simulink library "xpcseriallib"  (Simulink 7.7)
settings: Solver=FixedStepDiscrete  StartTime=0.0  StopTime=inf  RelTol=1e-3
undefined symbols (not defined in the file or in its folder): baddr1, baddr2, mbaseserialbinmask, mbaseserialmask, mdiamondemeraldfifomask, mdiamondemeraldmask, mmodemcontrol, mqua2mask, mquafifomask, mquamask, mrs232
libraries: xpcseriallib x614, xpclib x16, simulink x12
(part 1 of 7)
settings Model: Creator=gweast  LastModifiedBy=Darryl

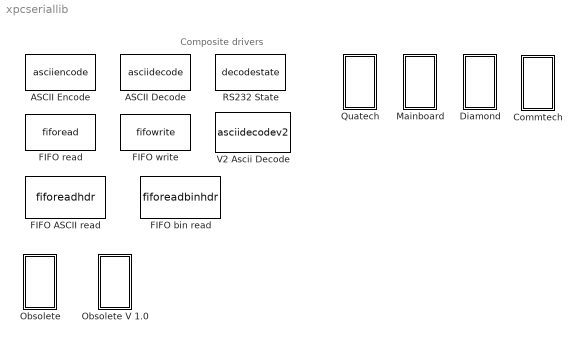
== system xpcseriallib ==
  note: Composite drivers
  "ASCII Decode " : S-Function  FunctionName=asciidecode  Parameters=format, nvars, varids  EnableBusSupport=off  mask(ASCII Decode){format=%d\\r, nvars=1, vartypes={ }}
      mask prompts: format "Format string:"; nvars "Number of variables:"; vartypes "Variable types:"
      mask help: ASCII decode -- Decode input string to output variables
      mask init:
      | [ maskdisplay, varids, format ] = masciidecode( 2, format, nvars, vartypes, 1 );
      | set_param( gcb, 'MaskDisplay', maskdisplay );
      mask Help: helpview(fullfile(docroot, 'mapfiles', 'xpc.map'), 'Quatech_ASCII_Decode')
      mask Display: disp( 'ASCII\nDecode');port_label('input',1,'D');port_label('output',1,'1');
  "ASCII Encode " : S-Function  FunctionName=asciiencode  Parameters=format, maxlength, nvars, varids  EnableBusSupport=off  mask(ASCII Encode){format=%d\\r, nvars=1, maxlength=128, vartypes={ 'double' }}
      mask prompts: format "Format string:"; nvars "Number of variables:"; maxlength "Max output string length:"; vartypes "Variable types:"
      mask help: ASCII Encode -- encode input variables as ascii for RS232.
      mask init:
      | [ maskdisplay, varids, format ] = masciidecode( 2, format, nvars, vartypes, 2 );
      | set_param( gcb, 'MaskDisplay', maskdisplay );
      mask Help: helpview(fullfile(docroot, 'mapfiles', 'xpc.map'), 'Quatech_ASCII_Encode')
      mask Display: disp( 'ASCII\nEncode');port_label('output',1,'D');port_label('input',1,'1');
  Commtech : Subsystem
      settings: OpenFcn=load_open_subsystem('xpccommtechlib',['xpccommtechlib/RS-422 &',char(10),'RS-485']);
  Diamond : Subsystem
  "FIFO ASCII read " : S-Function  FunctionName=fiforeadhdr  Parameters=maxsize, outputtype, sampletime, hdr, hlengths, nterm, hold, enable  EnableBusSupport=off  mask(Asynchronous FIFO Block: reader){header={'Header1','Header2'}, term=[13 10], hold=Zero output if no new data, enable=off, maxsize=1024, outputtype=8 bit uint null terminated, sampletime=0.01}
      mask prompts: term "Terminating string:"; hold "Output behavior:"; enable "Enable input:"; maxsize "Maximum read size:"; outputtype "Output vector type:"
      mask help: FIFO read multiple headers
      mask init:
      | [maskdisplay, hdr, hlengths, nterm] = mfiforhdr( header, term );
      | set_param( gcb, 'MaskDisplay', maskdisplay );
      mask Help: helpview(fullfile(docroot, 'mapfiles', 'xpc.map'), 'FIFO_asciiread')
      mask StyleString: edit,edit,popup(Hold last output if no new data|Zero output if no new data),checkbox,edit,popup(count+32 bit int|count+32 bit uint|count+16 bit int|count+16 bit uint|8 bit int null terminated|8 bit uint null terminated),edit
      mask Display: disp( 'FIFO\nRead HDRS');port_label('input',1,'F');port_label('output',1,'1');port_label('output',2,'2');
  "FIFO bin read " : S-Function  FunctionName=fiforeadbinhdr  Parameters=maxsize, outputtype, sampletime, hdr, hlengths, lengths, hold, enable  EnableBusSupport=off  mask(Asynchronous FIFO Block: reader){header={char([170, 1]), char([170,2])}, lengths=[3 4], hold=Zero output if no new data, enable=off, maxsize=1024, outputtype=8 bit uint null terminated, sampletime=0.01}
      mask prompts: lengths "Message Lengths:"; hold "Output behavior:"; enable "Enable input:"; maxsize "Maximum read size:"; outputtype "Output vector type:"
      mask help: FIFO read multiple binary headers
      mask init:
      | [maskdisplay, hdr, hlengths] = mfifobinhdr( header, lengths );
      | set_param( gcb, 'MaskDisplay', maskdisplay );
      mask Help: helpview(fullfile(docroot, 'mapfiles', 'xpc.map'), 'FIFO_binread')
      mask StyleString: edit,edit,popup(Hold last output if no new data|Zero output if no new data),checkbox,edit,popup(count+32 bit int|count+32 bit uint|count+16 bit int|count+16 bit uint|8 bit int null terminated|8 bit uint null terminated),edit
      mask Display: disp( 'FIFO\nRead BINARY');port_label('input',1,'F');port_label('output',1,'1');port_label('output',2,'2');
  "FIFO read " : S-Function  FunctionName=fiforead  Parameters=maxsize, minsize, usedelimiter, delimiter, outputtype, sampletime, enable, enableout  EnableBusSupport=off  mask(Asynchronous FIFO Block: reader){maxsize=1024, minsize=1, usedelimiter=on, delimiter=13, outputtype=8 bit uint null terminated, enable=off, enableout=off, sampletime=0.001}
      mask prompts: maxsize "Maximum read size:"; minsize "Minimum read size:"; usedelimiter "Read to delimiter:"; outputtype "Output vector type:"; enable "Max and Min read size ports:"; enableout "Enable passthrough:"
      mask help: FIFO read
      mask init:
      | maskdisplay = mfiforw( enable, enableout, 2 );
      | set_param( gcb, 'MaskDisplay', maskdisplay );
      mask Help: helpview(fullfile(docroot, 'mapfiles', 'xpc.map'), 'Quatech_FIFO_Read')
      mask StyleString: edit,edit,checkbox,edit,popup(count+32 bit int|count+32 bit uint|count+16 bit int|count+16 bit uint|8 bit int null terminated|8 bit uint null terminated),checkbox,checkbox,edit
      mask Display: disp( 'FIFO\nRead');port_label('output',1,'D');port_label('input',1,'F');
  "FIFO write " : S-Function  FunctionName=fifowrite  Parameters=size, inputtype, sampletime, present, id  EnableBusSupport=off  mask(Asynchronous FIFO Block: writer){size=1024, inputtype=8 bit uint null terminated, present=off, sampletime=-1, id=}
      mask prompts: inputtype "Input vector type:"; present "Data present output:"; id "ID (for overflow messages):"
      mask help: FIFO write
      mask init:
      | maskdisplay = mfiforw( present, 0, 1 );
      | set_param(gcb,'MaskDisplay',maskdisplay);
      mask Help: helpview(fullfile(docroot, 'mapfiles', 'xpc.map'), 'Quatech_FIFO_Write')
      mask StyleString: edit,popup(count+32 bit int|count+32 bit uint|count+16 bit int|count+16 bit uint|8 bit int null terminated|8 bit uint null terminated),checkbox,edit,edit
      mask Display: disp( 'FIFO\nwrite');port_label('input',1,'D');port_label('output', 1, 'F');
  Mainboard : Subsystem
  Obsolete : Subsystem
  Obsolete V 1.0 : Subsystem
  Quatech : Subsystem
  RS232 State : S-Function  FunctionName=decodestate  Parameters=overrun, parity, frame, breakint, count  EnableBusSupport=off  mask(RS232 State){overrun=on, parity=on, frame=off, breakint=off}
      mask prompts: overrun "Overrun error output:"; parity "Parity error output"; frame "Framing error output"; breakint "Break interrupt output"
      mask help: RS232 State
      mask init:
      | count = 0;
      | [maskdisplay, count] = mdecodestate( overrun, parity, frame, breakint );
      | set_param( gcb, 'MaskDisplay', maskdisplay );
      mask Help: helpview(fullfile(docroot, 'mapfiles', 'xpc.map'), 'Quatech_State')
      mask Display: disp('RS232\nState');port_label('input',1,'D');port_label('output',1,'D');port_label('output',2,'O');port_label('output',3,'P');
  "V2 Ascii Decode " : S-Function  FunctionName=asciidecodev2  Parameters=format, types  EnableBusSupport=off  mask(asciidecode2){format='%f\\n'}
      mask help: ASCII decode
      mask init:
      | [maskdisplay, types] = masciidecodev2( format );
      | set_param( gcb, 'MaskDisplay', maskdisplay );
      mask Help: helpview(fullfile(docroot, 'mapfiles', 'xpc.map'), 'ASCII_Decode2')
      mask Display: disp('Ascii Decode\nV2');port_label('output',1,'cnt');

== system xpcseriallib/Commtech ==

== system xpcseriallib/Diamond ==
  "Emerald-MM " : Subsystem
  "Emerald-MM8 " : Subsystem

== system xpcseriallib/Mainboard ==
  Baseboard Serial : Subsystem  InitFcn=mbaseserialmask(4,2);  mask(Baseboard RS232 Send Receive){group=Board Setup, port=1, irqnum=4, saddr1=0x3f8, saddr2=0x3e8, config=Com1/none, baud1=115200, parity1=None, ndata1=8, nstop1=1, fifomode1=16 deep, rlevel1=half full, automode1=off, xmtfifosize1=1024, xmtdatatype1=8 bit uint null terminated, rcvfifosize1=1024, rcvmaxread1=1024, rcvminread1=1, rcvusedelim1=on, rcvdelim1=13, rcvdatatype1=count+16 bit uint, rcvsampletime1=.01, baud2=115200, parity2=None, ndata2=8, nstop2=1, fifomode2=16 deep, rlevel2=half full, automode2=off, xmtfifosize2=1024, xmtdatatype2=8 bit uint null terminated, rcvfifosize2=1024, rcvmaxread2=1024, rcvminread2=1, rcvusedelim2=on, rcvdelim2=13, rcvdatatype2=count+16 bit uint, rcvsampletime2=.01}
      mask prompts: group "Parameter group:"; port "Port to modify:"; irqnum "IRQ number:"; saddr1 "First port address:"; saddr2 "Second port address:"; config "Configuration:"; baud1 "Baud rate:"; parity1 "Parity:"; ndata1 "Data bits:"; nstop1 "Stop bits:"; fifomode1 "Hardware FIFO size:"; rlevel1 "Receive FIFO interrupt level:"; automode1 "Auto RTS/CTS:"; xmtfifosize1 "Transmit software FIFO size:"; xmtdatatype1 "Transmit FIFO data type:"; rcvfifosize1 "Receive software FIFO size:"; rcvmaxread1 "Receive maximum read:"; rcvminread1 "Receive minimum read:"; rcvusedelim1 "Read to delimiter:"; rcvdelim1 "Delimiter:"; rcvdatatype1 "Receive data type:"; rcvsampletime1 "Receive SampleTime:"; baud2 "Baud rate:"; parity2 "Parity:"; ndata2 "Data bits:"; nstop2 "Stop bits:"; fifomode2 "Hardware FIFO size:"; rlevel2 "Receive FIFO interrupt level:"; automode2 "Auto RTS/CTS:"; xmtfifosize2 "Transmit software FIFO size:"; xmtdatatype2 "Transmit FIFO data type:"; rcvfifosize2 "Receive software fifo size:"; rcvmaxread2 "Receive maximum read:"; rcvminread2 "Receive minimum read:"; rcvusedelim2 "Read to delimiter:"; rcvdelim2 "Delimiter:"; rcvdatatype2 "Receive data type:"; rcvsampletime2 "Receive SampleTime:"
      mask help:
      | Baseboard
      | RS232 Send Receive Subsystem
      mask init:
      | [addr1, addr2, maskdisplay] = mbaseserialmask( 1, 2 );
      | baddr1 = addr1;
      | baddr2 = addr2;
      | mbaseserialmask( 3, 2 );
      | set_param( gcb, 'MaskDisplay', maskdisplay );
      mask Help: helpview(fullfile(docroot, 'mapfiles', 'xpc.map'), 'Baseboard_Serial_Subsystem')
      mask StyleString: popup(Board Setup|Basic Setup|Transmit Setup|Receive Setup),popup(1|2),edit,edit,edit,popup(Com1/none|Com2/none|Com1/Com3|Com2/Com4|none/Com3|none/Com4|Custom),popup(115200|57600|38400|19200|9600|4800|2400|1200|600|300|110),popup(None|Even|Odd|Mark|Space),popup(5|6|7|8),popup(1|2),popup(64 deep|16 deep|1 deep),popup(1|quarter full|half full|almost full),checkbox,edit,popup(count+32 bit int|count+32 bit uint|count+16 bit int|count+16 bit uint|8 bit int null terminated|8 bit uint null terminated),edit,edit,edit,checkbox,edit,popup(count+32 bit int|count+32 bit uint|count+16 bit int|count+16 bit uint|8 bit int null terminated|8 bit uint null terminated),edit,popup(115200|57600|38400|19200|9600|4800|2400|1200|600|300|110),popup(None|Even|Odd|Mark|Space),popup(5|6|7|8),popup(1|2),popup(64 deep|16 deep|1 deep),popup(1|quarter full|half full|almost full),checkbox,edit,popup(count+32 bit int|count+32 bit uint|count+16 bit int|count+16 bit uint|8 bit int null terminated|8 bit uint null terminated),edit,edit,edit,checkbox,edit,popup(count+32 bit int|count+32 bit uint|count+16 bit int|count+16 bit uint|8 bit int null terminated|8 bit uint null terminated),edit
      mask CallbackString:
      | mbaseserialmask( 2, 2 );
      | |mbaseserialmask( 2, 2 );||||mbaseserialmask( 2, 2 );
      | ||||||||||||||||||||||||||||||||
      mask Display: disp('Baseboard\nRS232\nSend Receive');port_label('input',1,'XMT1');port_label('input',2,'');port_label('output',1,'RCV1');port_label('output',2,'');
  Baseboard Serial Internal  blocks : Subsystem
  Baseboard Serial F : Subsystem  InitFcn=mbaseserialbinmask(4,2);  mask(Baseboard RS232 Send Receive){group=Board Setup, port=1, irqnum=4, saddr1=0x3f8, saddr2=0x3e8, config=Com1/none, baud1=115200, parity1=None, ndata1=8, nstop1=1, fifomode1=16 deep, rlevel1=half full, automode1=off, xmtfifosize1=1024, xmtdatatype1=8 bit uint null terminated, rcvfifosize1=1024, baud2=115200, parity2=None, ndata2=8, nstop2=1, fifomode2=16 deep, rlevel2=half full, automode2=off, xmtfifosize2=1024, xmtdatatype2=8 bit uint null terminated, rcvfifosize2=1024}
      mask prompts: group "Parameter group:"; port "Port to modify:"; irqnum "IRQ number:"; saddr1 "First port address:"; saddr2 "Second port address:"; config "Configuration:"; baud1 "Baud rate:"; parity1 "Parity:"; ndata1 "Data bits:"; nstop1 "Stop bits:"; fifomode1 "Hardware FIFO size:"; rlevel1 "Receive FIFO interrupt level:"; automode1 "Auto RTS/CTS:"; xmtfifosize1 "Transmit software FIFO size:"; xmtdatatype1 "Transmit FIFO data type:"; rcvfifosize1 "Receive software FIFO size:"; baud2 "Baud rate:"; parity2 "Parity:"; ndata2 "Data bits:"; nstop2 "Stop bits:"; fifomode2 "Hardware FIFO size:"; rlevel2 "Receive FIFO interrupt level:"; automode2 "Auto RTS/CTS:"; xmtfifosize2 "Transmit software FIFO size:"; xmtdatatype2 "Transmit FIFO data type:"; rcvfifosize2 "Receive software fifo size:"
      mask help:
      | Baseboard
      | RS232 Send Receive Subsystem
      mask init:
      | [addr1, addr2, maskdisplay] = mbaseserialbinmask( 1, 2 );
      | baddr1 = addr1;
      | baddr2 = addr2;
      | mbaseserialbinmask( 3, 2 );
      | set_param( gcb, 'MaskDisplay', maskdisplay );
      mask Help: helpview(fullfile(docroot, 'mapfiles', 'xpc.map'), 'Baseboard_Serial_Subsystem')
      mask StyleString: popup(Board Setup|Basic Setup|FIFO Setup),popup(1|2),edit,edit,edit,popup(Com1/none|Com2/none|Com1/Com3|Com2/Com4|none/Com3|none/Com4|Custom),popup(115200|57600|38400|19200|9600|4800|2400|1200|600|300|110),popup(None|Even|Odd|Mark|Space),popup(5|6|7|8),popup(1|2),popup(64 deep|16 deep|1 deep),popup(1|quarter full|half full|almost full),checkbox,edit,popup(count+32 bit int|count+32 bit uint|count+16 bit int|count+16 bit uint|8 bit int null terminated|8 bit uint null terminated),edit,popup(115200|57600|38400|19200|9600|4800|2400|1200|600|300|110),popup(None|Even|Odd|Mark|Space),popup(5|6|7|8),popup(1|2),popup(64 deep|16 deep|1 deep),popup(1|quarter full|half full|almost full),checkbox,edit,popup(count+32 bit int|count+32 bit uint|count+16 bit int|count+16 bit uint|8 bit int null terminated|8 bit uint null terminated),edit
      mask CallbackString:
      | mbaseserialbinmask( 2, 2 );
      | |mbaseserialbinmask( 2, 2 );||||mbaseserialbinmask( 2, 2 );
      | ||||||||||||||||||||
      mask Display: disp('Baseboard\nRS232\nSend Receive\nFIFO OUT');port_label('input',1,'XMT1');port_label('input',2,'');port_label('output',1,'FIFO1');port_label('output',2,'');
  Modem Control : S-Function  InitFcn=mmodemcontrol(4)  FunctionName=modemcontrolbase  Parameters=addr, boardtype, rts, dtr, count  EnableBusSupport=off  mask(Baseboard Modem Control){rts=on, dtr=on, config=Com1, addr=0x3f8}
      mask prompts: config "Configuration:"; addr "Base address:"
      mask help:
      | Baseboard
      | Modem Control
      mask init:
      | count = 0;
      | boardtype = 4;
      | [maskdisplay, count, addr] = mmodemcontrol( 2, rts, dtr, boardtype, config, addr );
      | addr = hex2dec( addr(3:end) );
      | set_param( gcb, 'MaskDisplay', maskdisplay );
      mask Help: helpview(fullfile(docroot, 'mapfiles', 'xpc.map'), 'Baseboard_MODEM_Control')
      mask StyleString: checkbox,checkbox,popup(Com1|Com2|Com3|Com4|Custom),edit
      mask CallbackString:
      | ||mmodemcontrol( 1 );
      | |
      mask Display: disp('Baseboard\nModem Control');port_label('input',1,'RTS');port_label('input',2,'DTR');
  Modem Status : S-Function  FunctionName=modemstatusbase  Parameters=addr, boardtype, cts, dsr, ring, dcd, count, sampletime  EnableBusSupport=off  mask(Modem Status){cts=on, dsr=on, ring=on, dcd=on, sampletime=-1, config=Com1, addr=0x3f8}
      mask prompts: ring "RI:"; config "Configuration:"; addr "Base address:"
      mask help:
      | Baseboard
      | Modem Status
      mask init:
      | count = 0;
      | boardtype = 4;
      | [maskdisplay, count, addr] = mmodemstatus( 2, cts, dsr, ring, dcd, boardtype, config, addr );
      | addr = hex2dec( addr(3:end) );
      | set_param( gcb, 'MaskDisplay', maskdisplay );
      mask Help: helpview(fullfile(docroot, 'mapfiles', 'xpc.map'), 'Baseboard_MODEM_Status')
      mask StyleString: checkbox,checkbox,checkbox,checkbox,edit,popup(Com1|Com2|Com3|Com4|Custom),edit
      mask CallbackString:
      | |||||mmodemstatus( 1 );
      | |
      mask Display: disp('Baseboard\nModem Status');port_label('output',1,'CTS');port_label('output',2,'DSR');port_label('output',3,'RI');port_label('output',4,'DCD');

== system xpcseriallib/Obsolete ==
  Asynchronous Mode : Subsystem
  Binary Mode : Subsystem
  "RS232 Setup " : S-Function  InitFcn=mrs232(0);  FunctionName=rs232setup  Parameters=port, baud, dbits, sbits, parity, prot, sbuf, rbuf, 0, istr, iack, iackto, tstr, tack, tackto, initinfo, initackinfo, terminfo, termackinfo  EnableBusSupport=off  mask(rs232setup){port=COM1, baud=9600, dbits=8, sbits=1, parity=None, prot=None, sbuf=1024, rbuf=1024, initstruct=[], termstruct=[]}
      mask prompts: baud "Baud rate:"; dbits "Number of data bits:"; sbits "Number of stop bits:"; prot "Protocol:"; sbuf "Send buffer size:"; rbuf "Receive buffer size:"; initstruct "Initialization command structure:"; termstruct "Termination command structure:"
      mask help:
      | RS-232
      | Mainboard
      | Setup
      mask init:
      | dmy = '';
      | [istr,iack,dmy,maskdisplay,maskdescription,dmy,dmy,dmy,dmy,initinfo,initackinfo,iackto]=mrs232(2,initstruct,4);
      | [tstr,tack,dmy,maskdisplay,maskdescription,dmy,dmy,dmy,dmy,terminfo,termackinfo,tackto]=mrs232(1,termstruct,4);
      | set_param(gcb,'MaskDisplay',maskdisplay);
      | set_param(gcb,'MaskDescription',maskdescription);
      mask Help: helpview(fullfile(docroot, 'mapfiles', 'xpc.map'), 'RS232_RS232')
      mask StyleString: popup(COM1|COM2|COM3|COM4),popup(115200|57600|38400|19200|9600|4800|2400|1200|600|300|110),popup(8|7),popup(1|2),popup(None|Odd|Even),popup(None|XOn XOff),edit,edit,edit,edit
      mask Display: disp('RS-232\nMainboard\nSetup');
  Synchronous Mode : Subsystem

== system xpcseriallib/Obsolete V 1.0 ==
  Asynchronous Mode : Subsystem
  "Setup " : Subsystem  mask(rs232setup){port=COM2, baudrate=115200, databit=8, stopbit=1, parity=None, protocol=None, sendbuf=1024, recbuf=1024}
      mask prompts: baudrate "Baud rate:"; databit "Number of data bits:"; stopbit "Number of stop bits:"; sendbuf "Send buffer size:"; recbuf "Receive buffer size:"
      mask help:
      | RS232 Kernel resident serial driver setup (Obsolete)
      | Version 1.0 compatible for backward compatibility
      | Not for use in new models
      mask Help: helpview(fullfile(docroot,'mapfiles','xpc.map'),'RS232_Setup');
      mask StyleString: popup(COM1|COM2|COM3|COM4),popup(115200|57600|38400|19200|9600|4800|2400|1200|300|110),popup(8|7|6|5),popup(1|2),popup(None|Odd|Even),popup(None|XOnXOff|RTSCTS|DTRDSR),edit,edit
      mask Display: disp('RS232\nMainboard\nSetup');
  Synchronous Mode : Subsystem

== system xpcseriallib/Quatech ==
  DSCP-200/300 : Subsystem
  ESC-100 : Subsystem
  QSC-100 : Subsystem
  QSC-200/300 : Subsystem

== system xpcseriallib/Diamond/Emerald-MM  ==
  Diamond Emerald-MM : Subsystem
  Diamond Emerald-MM Serial : Subsystem  InitFcn=mdiamondemeraldmask(4,4);  mask(Emerald-MM RS232 Send Receive){group=Board Setup, port=1, irqnum=7, saddr1=0x240, baud1=115200  (HS 460800), parity1=None, ndata1=8, nstop1=1, fifomode1=16 deep, rlevel1=half full, automode1=on, xmtfifosize1=1024, xmtdatatype1=8 bit uint null terminated, rcvfifosize1=1024, rcvmaxread1=1024, rcvminread1=1, rcvusedelim1=on, rcvdelim1=13, rcvdatatype1=count+16 bit uint, rcvsampletime1=-1, baud2=115200  (HS 460800), parity2=None, ndata2=8, nstop2=1, fifomode2=16 deep, rlevel2=half full, automode2=on, xmtfifosize2=1024, xmtdatatype2=8 bit uint null terminated, rcvfifosize2=1024, rcvmaxread2=1024, rcvminread2=1, rcvusedelim2=on, rcvdelim2=13, rcvdatatype2=count+16 bit uint, rcvsampletime2=-1, baud3=115200  (HS 460800), parity3=None, ndata3=8, nstop3=1, fifomode3=16 deep, rlevel3=half full, automode3=on, xmtfifosize3=1024, xmtdatatype3=8 bit uint null terminated, rcvfifosize3=1024, rcvmaxread3=1024, rcvminread3=1, rcvusedelim3=on, rcvdelim3=13, rcvdatatype3=count+16 bit uint, rcvsampletime3=-1, baud4=115200  (HS 460800), parity4=None, ndata4=8, nstop4=1, fifomode4=16 deep, rlevel4=half full, automode4=on, xmtfifosize4=1024, xmtdatatype4=8 bit uint null terminated, rcvfifosize4=1024, rcvmaxread4=1024, rcvminread4=1, rcvusedelim4=on, rcvdelim4=13, rcvdatatype4=count+16 bit uint, rcvsampletime4=-1}
      mask prompts: group "Parameter group:"; port "Port to modify:"; irqnum "IRQ number:"; saddr1 "First port address:"; baud1 "Baud rate:"; parity1 "Parity:"; ndata1 "Data bits:"; nstop1 "Stop bits:"; fifomode1 "Hardware FIFO size:"; rlevel1 "Receive FIFO interrupt level:"; automode1 "Auto RTS/CTS:"; xmtfifosize1 "Transmit software FIFO size:"; xmtdatatype1 "Transmit FIFO data type:"; rcvfifosize1 "Receive software FIFO size:"; rcvmaxread1 "Receive maximum read:"; rcvminread1 "Receive minimum read:"; rcvusedelim1 "Read to delimiter:"; rcvdelim1 "Delimiter:"; rcvdatatype1 "Receive data type:"; rcvsampletime1 "Receive SampleTime:"; baud2 "Baud rate:"; parity2 "Parity:"; ndata2 "Data bits:"; nstop2 "Stop bits:"; fifomode2 "Hardware FIFO size:"; rlevel2 "Receive FIFO interrupt level:"; automode2 "Auto RTS/CTS:"; xmtfifosize2 "Transmit software FIFO size:"; xmtdatatype2 "Transmit FIFO data type:"; rcvfifosize2 "Receive software FIFO size:"; rcvmaxread2 "Receive maximum read:"; rcvminread2 "Receive minimum read:"; rcvusedelim2 "Read to delimiter:"; rcvdelim2 "Delimiter:"; rcvdatatype2 "Receive data type:"; rcvsampletime2 "Receive SampleTime:"; baud3 "Baud rate:"; parity3 "Parity:"; ndata3 "Data bits:"; nstop3 "Stop bits:"; fifomode3 "Hardware FIFO size:"; rlevel3 "Receive FIFO interrupt level:"; automode3 "Auto RTS/CTS:"; xmtfifosize3 "Transmit software FIFO size:"; xmtdatatype3 "Transmit FIFO data type:"; rcvfifosize3 "Receive software FIFO size:"; rcvmaxread3 "Receive maximum read:"; rcvminread3 "Receive minimum read:"; rcvusedelim3 "Read to delimiter:"; rcvdelim3 "Delimiter:"; rcvdatatype3 "Receive data type:"; rcvsampletime3 "Receive SampleTime:"; baud4 "Baud rate:"; parity4 "Parity:"; ndata4 "Data bits:"; nstop4 "Stop bits:"; fifomode4 "Hardware FIFO size:"; rlevel4 "Receive FIFO interrupt level:"; automode4 "Auto RTS/CTS:"; xmtfifosize4 "Transmit software FIFO size:"; xmtdatatype4 "Transmit FIFO data type:"; rcvfifosize4 "Receive software FIFO size:"; rcvmaxread4 "Receive maximum read:"; rcvminread4 "Receive minimum read:"; rcvusedelim4 "Read to delimiter:"; rcvdelim4 "Delimiter:"; rcvdatatype4 "Receive data type:"; rcvsampletime4 "Receive SampleTime:"
      mask help:
      | Diamond Emerald
      | RS232 Send Receive Subsystem
      mask init:
      | addr = mdiamondemeraldmask( 1, 4 );
      | baddr1 = addr{1};
      | baddr2 = addr{2};
      | baddr3 = addr{3};
      | baddr4 = addr{4};
      | istat = addr{5};
      | mdiamondemeraldmask( 3, 4 );
      mask Help: helpview(fullfile(docroot, 'mapfiles', 'xpc.map'), 'Baseboard_Serial_Subsystem')
      mask StyleString: popup(Board Setup|Basic Setup|Transmit Setup|Receive Setup),popup(1|2|3|4),edit,popup(0x3F8|0x3E8|0x380|0x240|0x100|0x120|0x140|0x160),popup(115200  (HS 460800)|57600   (HS 230400)|38400   (HS 153600)|28800   (HS 115200)|19200   (HS 76800)|14400   (HS 57600)|9600    (HS 38400)|4800    (HS 19200)|2400    (HS 9600)|1200    (HS 4800)|600     (HS 2400)|300     (HS 1200)|150     (HS 600)|110     (HS 440)|75      (HS 300)|27.5    (HS 110)),popup(None|Even|Odd|Mark|Space),popup(5|6|7|8),popup(1|2),popup(64 deep|16 deep|1 deep),popup(1|quarter full|half full|almost full),checkbox,edit,popup(count+32 bit int|count+32 bit uint|count+16 bit int|count+16 bit uint|8 bit int null terminated|8 bit uint null terminated),edit,edit,edit,checkbox,edit,popup(count+32 bit int|count+32 bit uint|count+16 bit int|count+16 bit uint|8 bit int null terminated|8 bit uint null terminated),edit,popup(115200  (HS 460800)|57600   (HS 230400)|38400   (HS 153600)|28800   (HS 115200)|19200   (HS 76800)|14400   (HS 57600)|9600    (HS 38400)|4800    (HS 19200)|2400    (HS 9600)|1200    (HS 4800)|600     (HS 2400)|300     (HS 1200)|150     (HS 600)|110     (HS 440)|75      (HS 300)|27.5    (HS 110)),popup(None|Even|Odd|Mark|Space),popup(5|6|7|8),popup(1|2),popup(64 deep|16 deep|1 deep),popup(1|quarter full|half full|almost full),checkbox,edit,popup(count+32 bit int|count+32 bit uint|count+16 bit int|count+16 bit uint|8 bit int null terminated|8 bit uint null terminated),edit,edit,edit,checkbox,edit,popup(count+32 bit int|count+32 bit uint|count+16 bit int|count+16 bit uint|8 bit int null terminated|8 bit uint null terminated),edit,popup(115200  (HS 460800)|57600   (HS 230400)|38400   (HS 153600)|28800   (HS 115200)|19200   (HS 76800)|14400   (HS 57600)|9600    (HS 38400)|4800    (HS 19200)|2400    (HS 9600)|1200    (HS 4800)|600     (HS 2400)|300     (HS 1200)|150     (HS 600)|110     (HS 440)|75      (HS 300)|27.5    (HS 110)),popup(None|Even|Odd|Mark|Space),popup(5|6|7|8),popup(1|2),popup(64 deep|16 deep|1 deep),popup(1|quarter full|half full|almost full),checkbox,edit,popup(count+32 bit int|count+32 bit uint|count+16 bit int|count+16 bit uint|8 bit int null terminated|8 bit uint null terminated),edit,edit,edit,checkbox,edit,popup(count+32 bit int|count+32 bit uint|count+16 bit int|count+16 bit uint|8 bit int null terminated|8 bit uint null terminated),edit,popup(115200  (HS 460800)|57600   (HS 230400)|38400   (HS 153600)|28800   (HS 115200)|19200   (HS 76800)|14400   (HS 57600)|9600    (HS 38400)|4800    (HS 19200)|2400    (HS 9600)|1200    (HS 4800)|600     (HS 2400)|300     (HS 1200)|150     (HS 600)|110     (HS 440)|75      (HS 300)|27.5    (HS 110)),popup(None|Even|Odd|Mark|Space),popup(5|6|7|8),popup(1|2),popup(64 deep|16 deep|1 deep),popup(1|quarter full|half full|almost full),checkbox,edit,popup(count+32 bit int|count+32 bit uint|count+16 bit int|count+16 bit uint|8 bit int null terminated|8 bit uint null terminated),edit,edit,edit,checkbox,edit,popup(count+32 bit int|count+32 bit uint|count+16 bit int|count+16 bit uint|8 bit int null terminated|8 bit uint null terminated),edit
      mask CallbackString:
      | mdiamondemeraldmask( 2, 4 );
      | |mdiamondemeraldmask( 2, 4 );||||||||||||||||||||||||||||||||||||||||||||||||||||||||||||||||||
      mask Display:
      | disp('Diamond\n\nEmerald\nRS232\nSend Receive');
      | port_label('input',1,'XMT1');
      | port_label('input',2,'XMT2');
      | port_label('input',3,'XMT3');
      | port_label('input',4,'XMT4');
      | port_label('output',1,'RCV1');
      | port_label('output',2,'RCV2');
      | port_label('output',3,'RCV3');
      | port_label('output',4,'RCV4');
  Diamond Emerald-MM Serial F : Subsystem  InitFcn=mdiamondemeraldfifomask(4,4);  mask(Emerald-MM RS232 Send Receive){group=Board Setup, port=1, irqnum=7, saddr1=0x240, baud1=115200  (HS 460800), parity1=None, ndata1=8, nstop1=1, fifomode1=16 deep, rlevel1=half full, automode1=on, xmtfifosize1=1024, xmtdatatype1=8 bit uint null terminated, rcvfifosize1=1024, baud2=115200  (HS 460800), parity2=None, ndata2=8, nstop2=1, fifomode2=16 deep, rlevel2=half full, automode2=on, xmtfifosize2=1024, xmtdatatype2=8 bit uint null terminated, rcvfifosize2=1024, baud3=115200  (HS 460800), parity3=None, ndata3=8, nstop3=1, fifomode3=16 deep, rlevel3=half full, automode3=on, xmtfifosize3=1024, xmtdatatype3=8 bit uint null terminated, rcvfifosize3=1024, baud4=115200  (HS 460800), parity4=None, ndata4=8, nstop4=1, fifomode4=16 deep, rlevel4=half full, automode4=on, xmtfifosize4=1024, xmtdatatype4=8 bit uint null terminated, rcvfifosize4=1024}
      mask prompts: group "Parameter group:"; port "Port to modify:"; irqnum "IRQ number:"; saddr1 "First port address:"; baud1 "Baud rate:"; parity1 "Parity:"; ndata1 "Data bits:"; nstop1 "Stop bits:"; fifomode1 "Hardware FIFO size:"; rlevel1 "Receive FIFO interrupt level:"; automode1 "Auto RTS/CTS:"; xmtfifosize1 "Transmit software FIFO size:"; xmtdatatype1 "Transmit FIFO data type:"; rcvfifosize1 "Receive software FIFO size:"; baud2 "Baud rate:"; parity2 "Parity:"; ndata2 "Data bits:"; nstop2 "Stop bits:"; fifomode2 "Hardware FIFO size:"; rlevel2 "Receive FIFO interrupt level:"; automode2 "Auto RTS/CTS:"; xmtfifosize2 "Transmit software FIFO size:"; xmtdatatype2 "Transmit FIFO data type:"; rcvfifosize2 "Receive software FIFO size:"; baud3 "Baud rate:"; parity3 "Parity:"; ndata3 "Data bits:"; nstop3 "Stop bits:"; fifomode3 "Hardware FIFO size:"; rlevel3 "Receive FIFO interrupt level:"; automode3 "Auto RTS/CTS:"; xmtfifosize3 "Transmit software FIFO size:"; xmtdatatype3 "Transmit FIFO data type:"; rcvfifosize3 "Receive software FIFO size:"; baud4 "Baud rate:"; parity4 "Parity:"; ndata4 "Data bits:"; nstop4 "Stop bits:"; fifomode4 "Hardware FIFO size:"; rlevel4 "Receive FIFO interrupt level:"; automode4 "Auto RTS/CTS:"; xmtfifosize4 "Transmit software FIFO size:"; xmtdatatype4 "Transmit FIFO data type:"; rcvfifosize4 "Receive software FIFO size:"
      mask help:
      | Diamond Emerald
      | RS232 Send Receive Subsystem
      mask init:
      | addr = mdiamondemeraldfifomask( 1, 4 );
      | baddr1 = addr{1};
      | baddr2 = addr{2};
      | baddr3 = addr{3};
      | baddr4 = addr{4};
      | istat = addr{5};
      | mdiamondemeraldfifomask( 3, 4 );
      mask Help: helpview(fullfile(docroot, 'mapfiles', 'xpc.map'), 'Baseboard_Serial_Subsystem')
      mask StyleString: popup(Board Setup|Basic Setup|FIFO Setup),popup(1|2|3|4),edit,popup(0x3F8|0x3E8|0x380|0x240|0x100|0x120|0x140|0x160),popup(115200  (HS 460800)|57600   (HS 230400)|38400   (HS 153600)|28800   (HS 115200)|19200   (HS 76800)|14400   (HS 57600)|9600    (HS 38400)|4800    (HS 19200)|2400    (HS 9600)|1200    (HS 4800)|600     (HS 2400)|300     (HS 1200)|150     (HS 600)|110     (HS 440)|75      (HS 300)|27.5    (HS 110)),popup(None|Even|Odd|Mark|Space),popup(5|6|7|8),popup(1|2),popup(64 deep|16 deep|1 deep),popup(1|quarter full|half full|almost full),checkbox,edit,popup(count+32 bit int|count+32 bit uint|count+16 bit int|count+16 bit uint|8 bit int null terminated|8 bit uint null terminated),edit,popup(115200  (HS 460800)|57600   (HS 230400)|38400   (HS 153600)|28800   (HS 115200)|19200   (HS 76800)|14400   (HS 57600)|9600    (HS 38400)|4800    (HS 19200)|2400    (HS 9600)|1200    (HS 4800)|600     (HS 2400)|300     (HS 1200)|150     (HS 600)|110     (HS 440)|75      (HS 300)|27.5    (HS 110)),popup(None|Even|Odd|Mark|Space),popup(5|6|7|8),popup(1|2),popup(64 deep|16 deep|1 deep),popup(1|quarter full|half full|almost full),checkbox,edit,popup(count+32 bit int|count+32 bit uint|count+16 bit int|count+16 bit uint|8 bit int null terminated|8 bit uint null terminated),edit,popup(115200  (HS 460800)|57600   (HS 230400)|38400   (HS 153600)|28800   (HS 115200)|19200   (HS 76800)|14400   (HS 57600)|9600    (HS 38400)|4800    (HS 19200)|2400    (HS 9600)|1200    (HS 4800)|600     (HS 2400)|300     (HS 1200)|150     (HS 600)|110     (HS 440)|75      (HS 300)|27.5    (HS 110)),popup(None|Even|Odd|Mark|Space),popup(5|6|7|8),popup(1|2),popup(64 deep|16 deep|1 deep),popup(1|quarter full|half full|almost full),checkbox,edit,popup(count+32 bit int|count+32 bit uint|count+16 bit int|count+16 bit uint|8 bit int null terminated|8 bit uint null terminated),edit,popup(115200  (HS 460800)|57600   (HS 230400)|38400   (HS 153600)|28800   (HS 115200)|19200   (HS 76800)|14400   (HS 57600)|9600    (HS 38400)|4800    (HS 19200)|2400    (HS 9600)|1200    (HS 4800)|600     (HS 2400)|300     (HS 1200)|150     (HS 600)|110     (HS 440)|75      (HS 300)|27.5    (HS 110)),popup(None|Even|Odd|Mark|Space),popup(5|6|7|8),popup(1|2),popup(64 deep|16 deep|1 deep),popup(1|quarter full|half full|almost full),checkbox,edit,popup(count+32 bit int|count+32 bit uint|count+16 bit int|count+16 bit uint|8 bit int null terminated|8 bit uint null terminated),edit
      mask CallbackString:
      | mdiamondemeraldfifomask( 2, 4 );
      | |mdiamondemeraldfifomask( 2, 4 );||||||||||||||||||||||||||||||||||||||||||
      mask Display:
      | disp('Diamond\n\nEmerald\nRS232\n\nSend Receive\nFIFO OUT');
      | port_label('input',1,'XMT1');
      | port_label('input',2,'XMT2');
      | port_label('input',3,'XMT3');
      | port_label('input',4,'XMT4');
      | port_label('output',1,'FIFO1');
      | port_label('output',2,'FIFO2');
      | port_label('output',3,'FIFO3');
      | port_label('output',4,'FIFO4');
  "Modem Control " : S-Function  InitFcn=mmodemcontrol(5);  FunctionName=modemcontrolemeraldmm  Parameters=addr, boardtype, rts, dtr, count  EnableBusSupport=off  mask(Modem Control){port=1, rts=on, dtr=on, firstaddr=0x240}
      mask prompts: firstaddr "First port address:"
      mask help:
      | Diamond Emerald-MM
      | Modem Control
      mask init:
      | count = 0;
      | boardtype = 5;
      | [maskdisplay, count, addr] = mmodemcontrol( 2, rts, dtr, boardtype, port, firstaddr );
      | addr = hex2dec( addr(3:end) );
      | set_param( gcb, 'MaskDisplay', maskdisplay );
      mask Help: helpview(fullfile(docroot, 'mapfiles', 'xpc.map'), 'Emerald_MODEM_Control')
      mask StyleString: popup(1|2|3|4),checkbox,checkbox,popup(0x3F8|0x3E8|0x380|0x240|0x100|0x120|0x140)
      mask Display: disp('Diamond\nEmerald-MM\nModem Control');port_label('input',1,'RTS');port_label('input',2,'DTR');
  "Modem Status " : S-Function  FunctionName=modemstatusemeraldmm  Parameters=addr, boardtype, cts, dsr, ring, dcd, count, sampletime  EnableBusSupport=off  mask(Modem Status){port=1, cts=on, dsr=on, ring=on, dcd=on, sampletime=-1, firstaddr=0x240}
      mask prompts: ring "RI:"; firstaddr "First port address:"
      mask help:
      | Diamond Emerald-MM
      | Modem Status
      mask init:
      | count = 0;
      | boardtype = 5;
      | [maskdisplay, count, addr] = mmodemstatus( 2, cts, dsr, ring, dcd, boardtype, port, firstaddr );
      | addr = hex2dec( addr(3:end) );
      | set_param( gcb, 'MaskDisplay', maskdisplay );
      mask Help: helpview(fullfile(docroot, 'mapfiles', 'xpc.map'), 'Emerald_MODEM_Status')
      mask StyleString: popup(1|2|3|4),checkbox,checkbox,checkbox,checkbox,edit,popup(0x3F8|0x3E8|0x380|0x240|0x100|0x120|0x140)
      mask Display: disp('Diamond\nEmerald-MM\nModem Status');port_label('output',1,'CTS');port_label('output',2,'DSR');port_label('output',3,'RI');port_label('output',4,'DCD');
